simulink model "Exercise3"  (R2024b)
settings: Solver=VariableStepAuto  StartTime=0.0  StopTime=5400  FixedStep=1  MaxStep=5  RelTol=0.5e-5  AbsTol=1e-5
undefined symbols (not defined in the file): IAU, targetAmazon, targetNO
libraries: aerolibtransform2 x3, aerolibguid x2, slpidlib x1, sharedtransform x1, aerolibsatdyn x1, aerolibutil x1
settings Model: Creator=The MathWorks, Inc.  LastModifiedBy=jbrault
settings SolverCC: MaxConsecutiveMinStep=10  AutoInsertRateTranBlk=on  DecoupledContinuousIntegration=on  MinimalZcImpactIntegration=on  MaxZcPerStep=1
settings DataIOCC: DatasetSignalFormat=timetable  LoggingIntervals=[0, inf]
settings DebuggingCC: ReadBeforeWriteMsg=DisableAll  WriteAfterWriteMsg=DisableAll  WriteAfterReadMsg=DisableAll  MultiTaskDSMMsg=none  UnconnectedInputMsg=warning  UnconnectedOutputMsg=warning  UnconnectedLineMsg=warning
settings ModelReferenceCC: UpdateModelReferenceTargets=IfOutOfDate  EnableRefExpFcnMdlSchedulingChecks=on
settings SFSimCC: SFSimEcho=off
settings RTWCC: GPUComputeCapability=3.5  DLArmComputeVersion=19.05

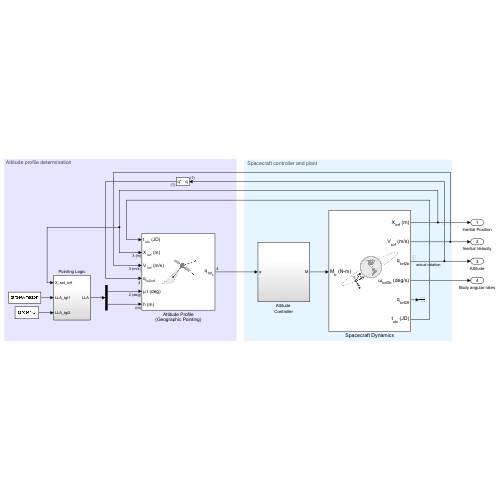
[thumbnail: Simulink's stored preview of the top-level diagram]
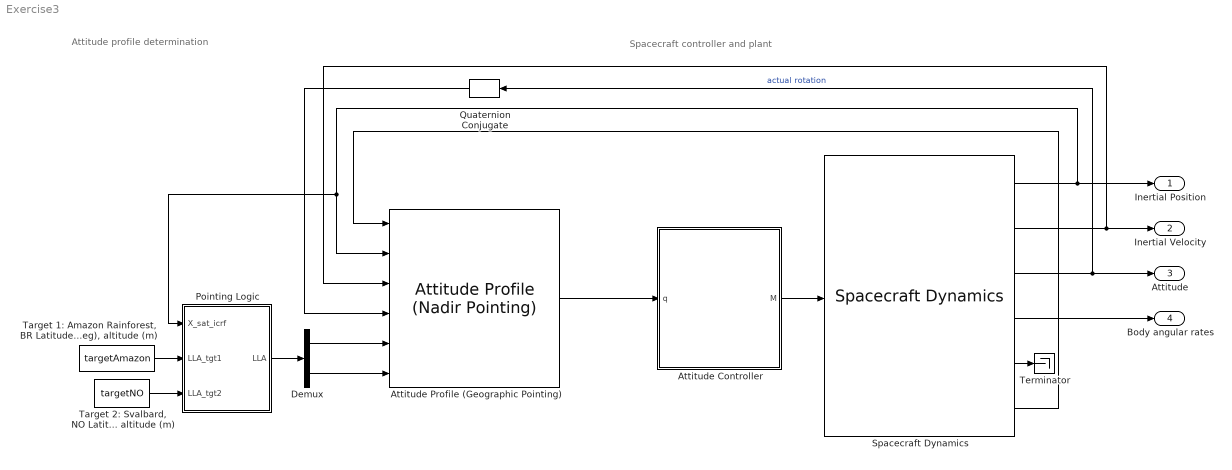
== system Exercise3 ==
  note: Attitude profile determination
  note: Spacecraft controller and plant
  Attitude Controller : Subsystem
  Attitude Profile (Geographic Pointing) : aerolibsatdyn/Attitude Profile (Nadir Pointing)  outputError=on  outputFinalAttitude=off  portFrame=ICRF  pointingMode=Point at LatLonAlt  celestialTarget=Sun  tunablePointing=off  primaryAlignmentSrc=Dialog  primaryAlignment=[0 0 1]  secondaryAlignmentSrc=Dialog  secondaryAlignment=[1 0 0]  constraintFrame=LVLH  primaryConstraintSrc=Dialog  primaryConstraint=[1 0 0]  secondaryConstraintSrc=Dialog  secondaryConstraint=[0 1 0]
  Demux : Demux  Outputs=[2 1]
  Pointing Logic : Subsystem
  Quaternion Conjugate : aerolibutil/Quaternion Conjugate
  Spacecraft Dynamics : SpacecraftDynamics  forcesIn=off  startDate=2459216  mass=1  inertia=eye(3)  semiMajorAxis=7200000  eccentricity=0.05  inclination=70  raan=215  argPeriapsis=0  trueAnomaly=200  attitude=[0.1509 0.4868 0.3031 -0.8052]  attitudeRate=[0 0 0]  outputTransform=on
  "Target 1: Amazon Rainforest, BR Latitude (deg), Longitude (deg), altitude (m)" : Constant  Value=targetAmazon
  "Target 2: Svalbard, NO Latitude (deg), Longitude (deg), altitude (m)" : Constant  Value=targetNO
  Terminator : Terminator
  Inertial Position : Outport
  Inertial Velocity : Outport  Port=2
  Attitude : Outport  Port=3
  Body angular rates : Outport  Port=4
  wires:
  Spacecraft Dynamics/2 -> Inertial Velocity/1, Attitude Profile (Geographic Pointing)/3
  Spacecraft Dynamics/1 -> Inertial Position/1, Pointing Logic/1(X_sat_icrf), Attitude Profile (Geographic Pointing)/2
  Spacecraft Dynamics/3 -> Attitude/1, Quaternion Conjugate/1  "actual rotation"
  Spacecraft Dynamics/6 -> Attitude Profile (Geographic Pointing)/1
  Attitude Profile (Geographic Pointing)/1 -> Attitude Controller/1(q)
  Attitude Controller/1(M) -> Spacecraft Dynamics/1
  Demux/1 -> Attitude Profile (Geographic Pointing)/5
  Demux/2 -> Attitude Profile (Geographic Pointing)/6
  Pointing Logic/1(LLA) -> Demux/1
  Quaternion Conjugate/1 -> Attitude Profile (Geographic Pointing)/4
  Spacecraft Dynamics/4 -> Body angular rates/1
  "Target 1: Amazon Rainforest, BR Latitude (deg), Longitude (deg), altitude (m)"/1 -> Pointing Logic/2(LLA_tgt1)
  "Target 2: Svalbard, NO Latitude (deg), Longitude (deg), altitude (m)"/1 -> Pointing Logic/3(LLA_tgt2)
  Spacecraft Dynamics/5 -> Terminator/1

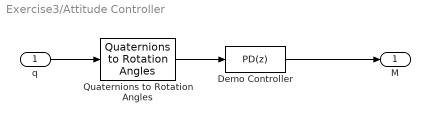
== system Exercise3/Attitude Controller ==
  q : Inport
  Demo Controller : slpidlib/PID Controller  Controller=PD  Form=Parallel  TimeDomain=Discrete-time  UseExternalTs=off  SampleTime=-1  IntegratorMethod=Trapezoidal  FilterMethod=Trapezoidal  ControllerParametersSource=internal  P=.000055  I=0  UseKiTs=off  D=.037  UseExternalDerivativeSource=off  N=1  UseFilter=off  TunerSelectOption=Transfer Function Based (PID Tuner App)  InitialConditionSource=internal  InitialConditionForIntegrator=0  InitialConditionForFilter=0  DifferentiatorICPrevScaledInput=0  ExternalReset=none  TrackingMode=off  Kt=1  LimitOutput=on  SatLimitsSource=internal  UpperSaturationLimit=0.008  LowerSaturationLimit=-0.008  LinearizeAsGain=on  AntiWindupMode=none  Kb=1  LimitIntegrator=off  UpperIntegratorSaturationLimit=inf  LowerIntegratorSaturationLimit=-inf  POutMin=[]  POutMax=[]  IOutMin=[]  IOutMax=[]  DOutMin=[]  DOutMax=[]  NOutMin=[]  NOutMax=[]  SumOutMin=[]  SumOutMax=[]  SaturationOutMin=[]  SaturationOutMax=[]  PParamMin=[]  PParamMax=[]  IParamMin=[]  IParamMax=[]  DParamMin=[]  DParamMax=[]  NParamMin=[]  NParamMax=[]  KbParamMin=[]  KbParamMax=[]  KtParamMin=[]  KtParamMax=[]  KbOutMin=[]  KbOutMax=[]  KtOutMin=[]  KtOutMax=[]  IntegratorOutMin=[]  IntegratorOutMax=[]  FilterOutMin=[]  FilterOutMax=[]  SumI1OutMin=[]  SumI1OutMax=[]  SumI2OutMin=[]  SumI2OutMax=[]  SumI3OutMin=[]  SumI3OutMax=[]  SumI4OutMin=[]  SumI4OutMax=[]  SumDOutMin=[]  SumDOutMax=[]  DifferentiatorOutMin=[]  DifferentiatorOutMax=[]  FilterDiffOutCoefMin=[]  FilterDiffOutCoefMax=[]  ReciprocalOutMin=[]  ReciprocalOutMax=[]  SumDenOutMin=[]  SumDenOutMax=[]  SumNumOutMin=[]  SumNumOutMax=[]  DivideOutMin=[]  DivideOutMax=[]  UdiffTsProdOutMin=[]  UdiffTsProdOutMax=[]  NTsProdOutMin=[]  NTsProdOutMax=[]  UintegralTsProdOutMin=[]  UintegralTsProdOutMax=[]  UngainTsProdOutMin=[]  UngainTsProdOutMax=[]  ClampingZeroOutDataTypeStr=Inherit: Inherit via back propagation  ClampingZeroOutMin=[]  ClampingZeroOutMax=[]  FilterDenConstantOutDataTypeStr=Inherit: Inherit via back propagation  FilterDenConstantOutMin=[]  FilterDenConstantOutMax=[]  PCopyOutDataTypeStr=Inherit: Inherit via back propagation  PCopyOutMin=[]  PCopyOutMax=[]  NCopyOutDataTypeStr=Inherit: Inherit via back propagation  NCopyOutMin=[]  NCopyOutMax=[]  IntegratorContinuousStateAttributes=''  IntegratorStateMustResolveToSignalObject=off  IntegratorRTWStateStorageClass=Auto  FilterContinuousStateAttributes=''  FilterStateMustResolveToSignalObject=off  FilterRTWStateStorageClass=Auto  ParallelPVariant=InternalParameters  IdealPVariant=Disabled  IVariant=Disabled  DVariant=InternalParameters  IntegratorVariant=Disabled  SatVariant=Enabled  AWVariant=Disabled  PCopyVariant=Disabled  TRVariant=Disabled  FdbkBlocksVariant=Forward  IdealPFdbkVariant=Disabled  SatFdbkVariant=Disabled  DerivativeFilterVariant=Differentiator  NVariant=Passthrough  NCopyVariant=Disabled_SignalSpec  FilterICVariant=InternalICsDifferentiator  IntegratorICVariant=Disabled  ExternalResetVariant=Disabled  TRSumVariant=Passthrough  SumFdbkVariant=Disabled  SumVariant=Sum_PD  TsampFilterVariant=InternalTs  TsampNgainVariant=Passthrough  TsampIntegralVariant=Disabled_SignalSpec  ExternalSaturationOutDataTypeStr=Inherit: Same as second input  DerivativeSourceVariant=ErrorSignal  PreIntVariant=InternalPreInt
  Quaternions to Rotation Angles : sharedtransform/Quaternions to Rotation Angles  rotationOrder=XYZ  aMode=aMode
  M : Outport
  wires:
  q/1 -> Quaternions to Rotation Angles/1
  Quaternions to Rotation Angles/1 -> Demo Controller/1
  Demo Controller/1 -> M/1

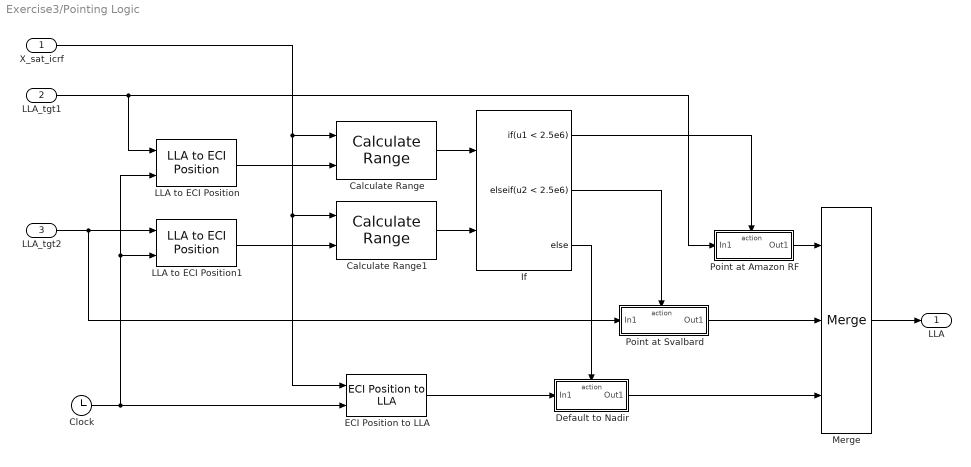
== system Exercise3/Pointing Logic ==
  X_sat_icrf : Inport
  LLA_tgt1 : Inport  Port=2
  LLA_tgt2 : Inport  Port=3
  Calculate Range : aerolibguid/Calculate Range
  Calculate Range1 : aerolibguid/Calculate Range
  Clock : Clock
  Default to Nadir : Subsystem  TreatAsAtomicUnit=on
  ECI Position to LLA : aerolibtransform2/ECI Position to LLA  red=IAU-2000/2006  year=2021  month=January  day=1  hour=12  min=0  sec=0  deltaT=Sec  errorflag=Error  extraparamflag=off  eunits=Metric (MKS)  earthmodel=WGS84  flat=1/298.257223563  eqradius=6378137
      settings: AttributesFormatString=%<red>
  If : If  NumInputs=2  IfExpression=u1 < 2.5e6  ElseIfExpressions=u2 < 2.5e6
  LLA to ECI Position : aerolibtransform2/LLA to ECI Position  red=IAU-2000/2006  year=2021  month=January  day=1  hour=12  min=0  sec=0  deltaT=Sec  errorflag=Error  extraparamflag=off  eunits=Metric (MKS)  earthmodel=WGS84  flat=1/298.257223563  eqradius=6378137
      settings: AttributesFormatString=%<red>
  LLA to ECI Position1 : aerolibtransform2/LLA to ECI Position  red=IAU-2000/2006  year=2021  month=January  day=1  hour=12  min=0  sec=0  deltaT=Sec  errorflag=Error  extraparamflag=off  eunits=Metric (MKS)  earthmodel=WGS84  flat=1/298.257223563  eqradius=6378137
      settings: AttributesFormatString=%<red>
  Merge : Merge  Inputs=3
  Point at Amazon RF : Subsystem  TreatAsAtomicUnit=on
  Point at Svalbard : Subsystem  TreatAsAtomicUnit=on
  LLA : Outport
  wires:
  ECI Position to LLA/1 -> Default to Nadir/1(In1)
  If/3 -> Default to Nadir/Action
  Default to Nadir/1(Out1) -> Merge/3
  Point at Amazon RF/1(Out1) -> Merge/1
  Merge/1 -> LLA/1
  LLA to ECI Position/1 -> Calculate Range/2
  If/1 -> Point at Amazon RF/Action
  If/2 -> Point at Svalbard/Action
  Point at Svalbard/1(Out1) -> Merge/2
  Calculate Range/1 -> If/1
  Calculate Range1/1 -> If/2
  LLA to ECI Position1/1 -> Calculate Range1/2
  LLA_tgt2/1 -> Point at Svalbard/1(In1), LLA to ECI Position1/1
  LLA_tgt1/1 -> Point at Amazon RF/1(In1), LLA to ECI Position/1
  X_sat_icrf/1 -> Calculate Range1/1, ECI Position to LLA/1, Calculate Range/1
  Clock/1 -> LLA to ECI Position/2, LLA to ECI Position1/2, ECI Position to LLA/2

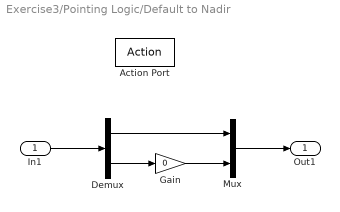
== system Exercise3/Pointing Logic/Default to Nadir ==
  In1 : Inport
  Action Port : ActionPort  ActionPortLabel=else
  Demux : Demux  Outputs=[2, 1]
  Gain : Gain  Gain=0
  Mux : Mux  Inputs=[2, 1]
  Out1 : Outport
  wires:
  In1/1 -> Demux/1
  Demux/1 -> Mux/1
  Demux/2 -> Gain/1
  Gain/1 -> Mux/2
  Mux/1 -> Out1/1

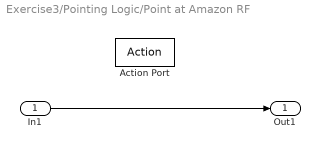
== system Exercise3/Pointing Logic/Point at Amazon RF ==
  In1 : Inport
  Action Port : ActionPort  ActionPortLabel=if(u1 < 2.5e6)
  Out1 : Outport
  wires:
  In1/1 -> Out1/1

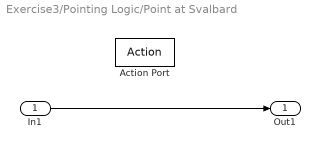
== system Exercise3/Pointing Logic/Point at Svalbard ==
  In1 : Inport
  Action Port : ActionPort  ActionPortLabel=elseif(u2 < 2.5e6)
  Out1 : Outport
  wires:
  In1/1 -> Out1/1
